simulink model "test2"  (R2018b)
settings: Solver=VariableStepAuto  StartTime=0.0  StopTime=50  RelTol=1e-3
values from neighbouring files (symbols this model uses):
  A = [0 1; 4 0]    [finally.m]    (also in q.m; test2.m)
  B = [1; 1]    [finally.m]    (also in q.m; test2.m)
  Bf = [2; 6]    [finally.m]    (also in q.m; test2.m)
  C = [3 0]    [finally.m]    (also in q.m; test2.m)
  D = 3    [finally.m]    (also in q.m; test2.m)
  Gg = [0 1; 0 0]    [finally.m]    (also in test2.m)
  Hg = [1 0]    [finally.m]    (also in q.m; test2.m)
  K = [K_(2) K_(3)]    [test2.m]
  Kl = K_(1)    [test2.m]
  Mg = [m11Sol m12Sol; m21Sol m22Sol]    [test2.m]
settings Model: Creator=kekos  LastModifiedBy=kekos

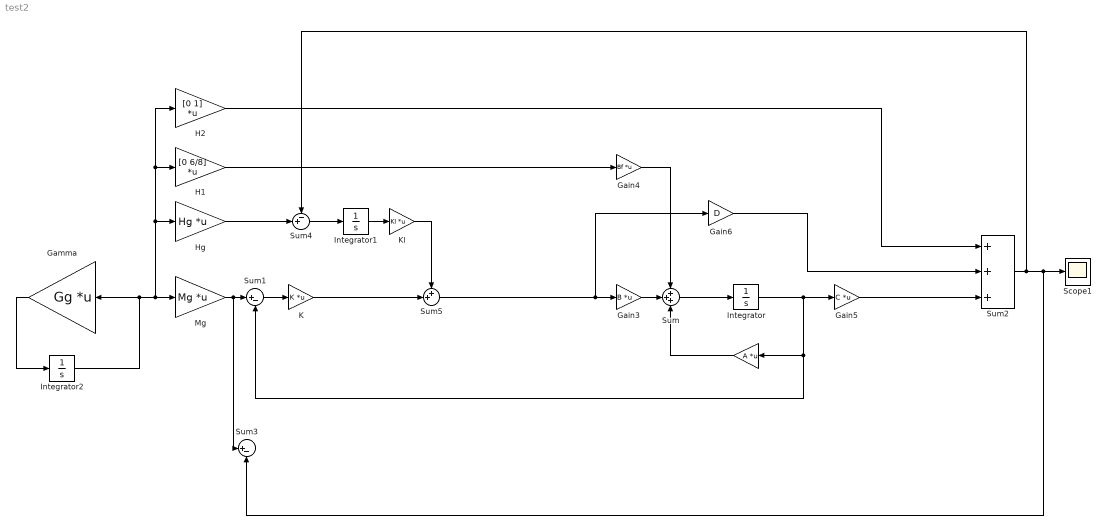
== system test2 ==
  " " : Gain  Gain=A  Multiplication=Matrix(K*u)
  Gain3 : Gain  Gain=B  Multiplication=Matrix(K*u)
  Gain4 : Gain  Gain=Bf  Multiplication=Matrix(K*u)
  Gain5 : Gain  Gain=C  Multiplication=Matrix(K*u)
  Gain6 : Gain  Gain=D
  Gamma : Gain  Gain=Gg  Multiplication=Matrix(K*u)
  H1 : Gain  Gain=[0 6/8]  Multiplication=Matrix(K*u)
  H2 : Gain  Gain=[0 1]  Multiplication=Matrix(K*u)
  Hg : Gain  Gain=Hg  Multiplication=Matrix(K*u)
  Integrator : Integrator
  Integrator1 : Integrator
  Integrator2 : Integrator  InitialCondition=[0; 8]
  K : Gain  Gain=K  Multiplication=Matrix(K*u)
  Kl : Gain  Gain=Kl  Multiplication=Matrix(K*u)
  Mg : Gain  Gain=Mg  Multiplication=Matrix(K*u)
  Scope1 : Scope
  Sum : Sum  Inputs=+++
  Sum1 : Sum  Inputs=|+-
  Sum2 : Sum  Inputs=+++
  Sum3 : Sum  Inputs=|+-
  Sum4 : Sum  Inputs=-+|
  Sum5 : Sum  Inputs=++|
  wires:
  Gain4/1 -> Sum/1
  Gamma/1 -> Integrator2/1
  H2/1 -> Sum2/1
  Gain6/1 -> Sum2/2
  Sum5/1 -> Gain6/1, Gain3/1
  Gain3/1 -> Sum/2
  " "/1 -> Sum/3
  Integrator/1 -> Gain5/1, " "/1, Sum1/2
  Integrator2/1 -> Mg/1, Hg/1, H2/1, H1/1, Gamma/1
  Gain5/1 -> Sum2/3
  H1/1 -> Gain4/1
  Sum1/1 -> K/1
  Sum/1 -> Integrator/1
  Sum2/1 -> Sum3/2, Scope1/1, Sum4/1
  Mg/1 -> Sum3/1, Sum1/1
  K/1 -> Sum5/2
  Hg/1 -> Sum4/2
  Sum4/1 -> Integrator1/1
  Integrator1/1 -> Kl/1
  Kl/1 -> Sum5/1
